simulink model "DiagCCaller_TestHarness"  (R2019a)
settings: Solver=FixedStepDiscrete  StartTime=0.0  StopTime=10.0  FixedStep=0.1  RelTol=1e-3  EnableMultiTasking=on
undefined symbols (not defined in the file): Dem_EventStatusType, sigbuilder_block
(part 2 of 4)

== system DiagCCaller_TestHarness/Debounce Enabled - RESET by Disable\Enable subsystem,Fault Active, FaultCnt = 10, PassCnt = -5, Heal 1  ==
  Bus Creator : BusCreator  Inputs=15
  Data Type Conversion{,1..2,9..14} (9 alike) : DataTypeConversion  OutDataTypeStr=boolean
  Data Type Conversion3 : DataTypeConversion  OutDataTypeStr=single
  Data Type Conversion4 : DataTypeConversion  OutDataTypeStr=single
  Data Type Conversion{5..8} (4 alike) : DataTypeConversion  OutDataTypeStr=int16
  Signal Builder : Subsystem  Tag=STV Subsys  LoadFcn=sigbuilder_block('load');  StartFcn=sigbuilder_block('start');  StopFcn=sigbuilder_block('stop');  ClipboardFcn=sigbuilder_block('clipboard');  TreatAsAtomicUnit=on  mask(Sigbuilder block){tuvar=[0:10]}
      mask help: Simulink:masks:SigbuilderBlock_MD
      mask init:
      | if ~strcmp(get_param(bdroot(gcbh),'SimulationStatus'),'stopped') tuvar = sigbuilder_block('maskInit'); end
      settings: CopyFcn=sigbuilder_block('copy');  DeleteFcn=sigbuilder_block('delete');  ModelCloseFcn=sigbuilder_block('modelClose');  PreSaveFcn=sigbuilder_block('preSave');  PauseFcn=sigbuilder_block('pause');  ContinueFcn=sigbuilder_block('continue');  NameChangeFcn=sigbuilder_block('namechange');  OpenFcn=sigbuilder_block('open',[5.4 30 1141.2 522.6 ]);  CloseFcn=sigbuilder_block('close');
      mask Display: plot(0, 0, 100, 100,[2, 2, 32, 32, 2], [68, 8, 8, 68, 68],[32, 2], [38, 38], [32, 19, 2],[53, 60, 44], [32, 17, 17, 2],[16, 16, 31, 31]);txt = getActiveGroup(gcbh);text(2, 100, txt,'verticalAlignment', 'top');
  Out1 : Outport
  wires:
  Bus Creator/1 -> Out1/1
  Signal Builder/2(DiagInput) -> Data Type Conversion1/1
  Signal Builder/3(StartupComp) -> Data Type Conversion2/1
  Signal Builder/4(MaxValue) -> Data Type Conversion4/1
  Signal Builder/5(MinValue) -> Data Type Conversion3/1
  Signal Builder/6(UpCount) -> Data Type Conversion5/1
  Signal Builder/7(DownCount) -> Data Type Conversion6/1
  Signal Builder/8(FaultCountThd) -> Data Type Conversion7/1
  Signal Builder/9(PassCountThd) -> Data Type Conversion8/1
  Signal Builder/10(DebounceEn) -> Data Type Conversion9/1
  Signal Builder/11(DiagReset) -> Data Type Conversion10/1
  Signal Builder/12(DiagEnable) -> Data Type Conversion11/1
  Signal Builder/13(HealEnable) -> Data Type Conversion12/1
  Signal Builder/14(PreestorageFreezeTrigger) -> Data Type Conversion13/1
  Signal Builder/15(JumpDownEn) -> Data Type Conversion14/1
  Signal Builder/1(EnableSubsystem) -> Data Type Conversion/1
  Data Type Conversion/1 -> Bus Creator/1  "EnableSubsystem"
  Data Type Conversion1/1 -> Bus Creator/2  "DiagInput"
  Data Type Conversion2/1 -> Bus Creator/3  "StartupComp"
  Data Type Conversion4/1 -> Bus Creator/4  "MaxValue"
  Data Type Conversion3/1 -> Bus Creator/5  "MinValue"
  Data Type Conversion5/1 -> Bus Creator/6  "UpCount"
  Data Type Conversion6/1 -> Bus Creator/7  "DownCount"
  Data Type Conversion7/1 -> Bus Creator/8  "FaultCountThd"
  Data Type Conversion8/1 -> Bus Creator/9  "PassCountThd"
  Data Type Conversion9/1 -> Bus Creator/10  "DebounceEn"
  Data Type Conversion10/1 -> Bus Creator/11  "DiagReset"
  Data Type Conversion11/1 -> Bus Creator/12  "DiagEnable"
  Data Type Conversion12/1 -> Bus Creator/13  "HealEnable"
  Data Type Conversion13/1 -> Bus Creator/14  "PreestorageFreezeTrigger"
  Data Type Conversion14/1 -> Bus Creator/15  "JumpDownEn"

== system DiagCCaller_TestHarness/Debounce Enabled - RESET by Disable\Enable subsystem,Fault Active, FaultCnt = 10, PassCnt = 0 , Heal 0  ==
  Bus Creator : BusCreator  Inputs=15
  Data Type Conversion{,1..2,9..14} (9 alike) : DataTypeConversion  OutDataTypeStr=boolean
  Data Type Conversion3 : DataTypeConversion  OutDataTypeStr=single
  Data Type Conversion4 : DataTypeConversion  OutDataTypeStr=single
  Data Type Conversion{5..8} (4 alike) : DataTypeConversion  OutDataTypeStr=int16
  Signal Builder : Subsystem  Tag=STV Subsys  LoadFcn=sigbuilder_block('load');  StartFcn=sigbuilder_block('start');  StopFcn=sigbuilder_block('stop');  ClipboardFcn=sigbuilder_block('clipboard');  TreatAsAtomicUnit=on  mask(Sigbuilder block){tuvar=[0:10]}
      mask help: Simulink:masks:SigbuilderBlock_MD
      mask init:
      | if ~strcmp(get_param(bdroot(gcbh),'SimulationStatus'),'stopped') tuvar = sigbuilder_block('maskInit'); end
      settings: CopyFcn=sigbuilder_block('copy');  DeleteFcn=sigbuilder_block('delete');  ModelCloseFcn=sigbuilder_block('modelClose');  PreSaveFcn=sigbuilder_block('preSave');  PauseFcn=sigbuilder_block('pause');  ContinueFcn=sigbuilder_block('continue');  NameChangeFcn=sigbuilder_block('namechange');  OpenFcn=sigbuilder_block('open',[5.4 5.4 1141.2 580.8 ]);  CloseFcn=sigbuilder_block('close');
      mask Display: plot(0, 0, 100, 100,[2, 2, 32, 32, 2], [68, 8, 8, 68, 68],[32, 2], [38, 38], [32, 19, 2],[53, 60, 44], [32, 17, 17, 2],[16, 16, 31, 31]);txt = getActiveGroup(gcbh);text(2, 100, txt,'verticalAlignment', 'top');
  Out1 : Outport
  wires:
  Data Type Conversion14/1 -> Bus Creator/15  "JumpDownEn"
  Data Type Conversion13/1 -> Bus Creator/14  "PreestorageFreezeTrigger"
  Data Type Conversion12/1 -> Bus Creator/13  "HealEnable"
  Data Type Conversion11/1 -> Bus Creator/12  "DiagEnable"
  Data Type Conversion10/1 -> Bus Creator/11  "DiagReset"
  Data Type Conversion9/1 -> Bus Creator/10  "DebounceEn"
  Data Type Conversion8/1 -> Bus Creator/9  "PassCountThd"
  Data Type Conversion7/1 -> Bus Creator/8  "FaultCountThd"
  Data Type Conversion6/1 -> Bus Creator/7  "DownCount"
  Data Type Conversion5/1 -> Bus Creator/6  "UpCount"
  Data Type Conversion3/1 -> Bus Creator/5  "MinValue"
  Data Type Conversion4/1 -> Bus Creator/4  "MaxValue"
  Data Type Conversion2/1 -> Bus Creator/3  "StartupComp"
  Data Type Conversion1/1 -> Bus Creator/2  "DiagInput"
  Data Type Conversion/1 -> Bus Creator/1  "EnableSubsystem"
  Signal Builder/1(EnableSubsystem) -> Data Type Conversion/1
  Signal Builder/15(JumpDownEn) -> Data Type Conversion14/1
  Signal Builder/14(PreestorageFreezeTrigger) -> Data Type Conversion13/1
  Signal Builder/13(HealEnable) -> Data Type Conversion12/1
  Signal Builder/12(DiagEnable) -> Data Type Conversion11/1
  Signal Builder/11(DiagReset) -> Data Type Conversion10/1
  Signal Builder/10(DebounceEn) -> Data Type Conversion9/1
  Signal Builder/9(PassCountThd) -> Data Type Conversion8/1
  Signal Builder/8(FaultCountThd) -> Data Type Conversion7/1
  Signal Builder/7(DownCount) -> Data Type Conversion6/1
  Signal Builder/6(UpCount) -> Data Type Conversion5/1
  Signal Builder/5(MinValue) -> Data Type Conversion3/1
  Signal Builder/4(MaxValue) -> Data Type Conversion4/1
  Signal Builder/3(StartupComp) -> Data Type Conversion2/1
  Signal Builder/2(DiagInput) -> Data Type Conversion1/1
  Bus Creator/1 -> Out1/1

== system DiagCCaller_TestHarness/Debounce Enabled - RESET by Disable\Enable subsystem,Fault Inactive,  FaultCnt = 10, PassCnt = -5 , Heal 1  ==
  Bus Creator : BusCreator  Inputs=15
  Data Type Conversion{,1..2,9..14} (9 alike) : DataTypeConversion  OutDataTypeStr=boolean
  Data Type Conversion3 : DataTypeConversion  OutDataTypeStr=single
  Data Type Conversion4 : DataTypeConversion  OutDataTypeStr=single
  Data Type Conversion{5..8} (4 alike) : DataTypeConversion  OutDataTypeStr=int16
  Signal Builder : Subsystem  Tag=STV Subsys  LoadFcn=sigbuilder_block('load');  StartFcn=sigbuilder_block('start');  StopFcn=sigbuilder_block('stop');  ClipboardFcn=sigbuilder_block('clipboard');  TreatAsAtomicUnit=on  mask(Sigbuilder block){tuvar=[0:10]}
      mask help: Simulink:masks:SigbuilderBlock_MD
      mask init:
      | if ~strcmp(get_param(bdroot(gcbh),'SimulationStatus'),'stopped') tuvar = sigbuilder_block('maskInit'); end
      settings: CopyFcn=sigbuilder_block('copy');  DeleteFcn=sigbuilder_block('delete');  ModelCloseFcn=sigbuilder_block('modelClose');  PreSaveFcn=sigbuilder_block('preSave');  PauseFcn=sigbuilder_block('pause');  ContinueFcn=sigbuilder_block('continue');  NameChangeFcn=sigbuilder_block('namechange');  OpenFcn=sigbuilder_block('open',[1440 -222 1440 813.6 ]);  CloseFcn=sigbuilder_block('close');
      mask Display: plot(0, 0, 100, 100,[2, 2, 32, 32, 2], [68, 8, 8, 68, 68],[32, 2], [38, 38], [32, 19, 2],[53, 60, 44], [32, 17, 17, 2],[16, 16, 31, 31]);txt = getActiveGroup(gcbh);text(2, 100, txt,'verticalAlignment', 'top');
  Out1 : Outport
  wires:
  Data Type Conversion14/1 -> Bus Creator/15  "JumpDownEn"
  Data Type Conversion13/1 -> Bus Creator/14  "PreestorageFreezeTrigger"
  Data Type Conversion12/1 -> Bus Creator/13  "HealEnable"
  Data Type Conversion11/1 -> Bus Creator/12  "DiagEnable"
  Data Type Conversion10/1 -> Bus Creator/11  "DiagReset"
  Data Type Conversion9/1 -> Bus Creator/10  "DebounceEn"
  Data Type Conversion8/1 -> Bus Creator/9  "PassCountThd"
  Data Type Conversion7/1 -> Bus Creator/8  "FaultCountThd"
  Data Type Conversion6/1 -> Bus Creator/7  "DownCount"
  Data Type Conversion5/1 -> Bus Creator/6  "UpCount"
  Data Type Conversion3/1 -> Bus Creator/5  "MinValue"
  Data Type Conversion4/1 -> Bus Creator/4  "MaxValue"
  Data Type Conversion2/1 -> Bus Creator/3  "StartupComp"
  Data Type Conversion1/1 -> Bus Creator/2  "DiagInput"
  Data Type Conversion/1 -> Bus Creator/1  "EnableSubsystem"
  Signal Builder/1(EnableSubsystem) -> Data Type Conversion/1
  Signal Builder/15(JumpDownEn) -> Data Type Conversion14/1
  Signal Builder/14(PreestorageFreezeTrigger) -> Data Type Conversion13/1
  Signal Builder/13(HealEnable) -> Data Type Conversion12/1
  Signal Builder/12(DiagEnable) -> Data Type Conversion11/1
  Signal Builder/11(DiagReset) -> Data Type Conversion10/1
  Signal Builder/10(DebounceEn) -> Data Type Conversion9/1
  Signal Builder/9(PassCountThd) -> Data Type Conversion8/1
  Signal Builder/8(FaultCountThd) -> Data Type Conversion7/1
  Signal Builder/7(DownCount) -> Data Type Conversion6/1
  Signal Builder/6(UpCount) -> Data Type Conversion5/1
  Signal Builder/5(MinValue) -> Data Type Conversion3/1
  Signal Builder/4(MaxValue) -> Data Type Conversion4/1
  Signal Builder/3(StartupComp) -> Data Type Conversion2/1
  Signal Builder/2(DiagInput) -> Data Type Conversion1/1
  Bus Creator/1 -> Out1/1

== system DiagCCaller_TestHarness/Debounce Enabled - RESET by Disable\Enable subsystem,Fault Inactive, , FaultCnt = 10, PassCnt = 0 , Heal 0  ==
  Bus Creator : BusCreator  Inputs=15
  Data Type Conversion{,1..2,9..14} (9 alike) : DataTypeConversion  OutDataTypeStr=boolean
  Data Type Conversion3 : DataTypeConversion  OutDataTypeStr=single
  Data Type Conversion4 : DataTypeConversion  OutDataTypeStr=single
  Data Type Conversion{5..8} (4 alike) : DataTypeConversion  OutDataTypeStr=int16
  Signal Builder : Subsystem  Tag=STV Subsys  LoadFcn=sigbuilder_block('load');  StartFcn=sigbuilder_block('start');  StopFcn=sigbuilder_block('stop');  ClipboardFcn=sigbuilder_block('clipboard');  TreatAsAtomicUnit=on  mask(Sigbuilder block){tuvar=[0:10]}
      mask help: Simulink:masks:SigbuilderBlock_MD
      mask init:
      | if ~strcmp(get_param(bdroot(gcbh),'SimulationStatus'),'stopped') tuvar = sigbuilder_block('maskInit'); end
      settings: CopyFcn=sigbuilder_block('copy');  DeleteFcn=sigbuilder_block('delete');  ModelCloseFcn=sigbuilder_block('modelClose');  PreSaveFcn=sigbuilder_block('preSave');  PauseFcn=sigbuilder_block('pause');  ContinueFcn=sigbuilder_block('continue');  NameChangeFcn=sigbuilder_block('namechange');  OpenFcn=sigbuilder_block('open',[5.4 30 1141.2 522.6 ]);  CloseFcn=sigbuilder_block('close');
      mask Display: plot(0, 0, 100, 100,[2, 2, 32, 32, 2], [68, 8, 8, 68, 68],[32, 2], [38, 38], [32, 19, 2],[53, 60, 44], [32, 17, 17, 2],[16, 16, 31, 31]);txt = getActiveGroup(gcbh);text(2, 100, txt,'verticalAlignment', 'top');
  Out1 : Outport
  wires:
  Data Type Conversion14/1 -> Bus Creator/15  "JumpDownEn"
  Data Type Conversion13/1 -> Bus Creator/14  "PreestorageFreezeTrigger"
  Data Type Conversion12/1 -> Bus Creator/13  "HealEnable"
  Data Type Conversion11/1 -> Bus Creator/12  "DiagEnable"
  Data Type Conversion10/1 -> Bus Creator/11  "DiagReset"
  Data Type Conversion9/1 -> Bus Creator/10  "DebounceEn"
  Data Type Conversion8/1 -> Bus Creator/9  "PassCountThd"
  Data Type Conversion7/1 -> Bus Creator/8  "FaultCountThd"
  Data Type Conversion6/1 -> Bus Creator/7  "DownCount"
  Data Type Conversion5/1 -> Bus Creator/6  "UpCount"
  Data Type Conversion3/1 -> Bus Creator/5  "MinValue"
  Data Type Conversion4/1 -> Bus Creator/4  "MaxValue"
  Data Type Conversion2/1 -> Bus Creator/3  "StartupComp"
  Data Type Conversion1/1 -> Bus Creator/2  "DiagInput"
  Data Type Conversion/1 -> Bus Creator/1  "EnableSubsystem"
  Signal Builder/1(EnableSubsystem) -> Data Type Conversion/1
  Signal Builder/15(JumpDownEn) -> Data Type Conversion14/1
  Signal Builder/14(PreestorageFreezeTrigger) -> Data Type Conversion13/1
  Signal Builder/13(HealEnable) -> Data Type Conversion12/1
  Signal Builder/12(DiagEnable) -> Data Type Conversion11/1
  Signal Builder/11(DiagReset) -> Data Type Conversion10/1
  Signal Builder/10(DebounceEn) -> Data Type Conversion9/1
  Signal Builder/9(PassCountThd) -> Data Type Conversion8/1
  Signal Builder/8(FaultCountThd) -> Data Type Conversion7/1
  Signal Builder/7(DownCount) -> Data Type Conversion6/1
  Signal Builder/6(UpCount) -> Data Type Conversion5/1
  Signal Builder/5(MinValue) -> Data Type Conversion3/1
  Signal Builder/4(MaxValue) -> Data Type Conversion4/1
  Signal Builder/3(StartupComp) -> Data Type Conversion2/1
  Signal Builder/2(DiagInput) -> Data Type Conversion1/1
  Bus Creator/1 -> Out1/1

== system DiagCCaller_TestHarness/Debounce Enabled - RESET by Disable\Enable subsystem,Fault Inactive, , FaultCnt = 10, PassCnt = 0 , Heal 0 1 ==
  Bus Creator : BusCreator  Inputs=15
  Data Type Conversion{,1..2,9..14} (9 alike) : DataTypeConversion  OutDataTypeStr=boolean
  Data Type Conversion3 : DataTypeConversion  OutDataTypeStr=single
  Data Type Conversion4 : DataTypeConversion  OutDataTypeStr=single
  Data Type Conversion{5..8} (4 alike) : DataTypeConversion  OutDataTypeStr=int16
  Signal Builder : Subsystem  Tag=STV Subsys  LoadFcn=sigbuilder_block('load');  StartFcn=sigbuilder_block('start');  StopFcn=sigbuilder_block('stop');  ClipboardFcn=sigbuilder_block('clipboard');  TreatAsAtomicUnit=on  mask(Sigbuilder block){tuvar=[0:10]}
      mask help: Simulink:masks:SigbuilderBlock_MD
      mask init:
      | if ~strcmp(get_param(bdroot(gcbh),'SimulationStatus'),'stopped') tuvar = sigbuilder_block('maskInit'); end
      settings: CopyFcn=sigbuilder_block('copy');  DeleteFcn=sigbuilder_block('delete');  ModelCloseFcn=sigbuilder_block('modelClose');  PreSaveFcn=sigbuilder_block('preSave');  PauseFcn=sigbuilder_block('pause');  ContinueFcn=sigbuilder_block('continue');  NameChangeFcn=sigbuilder_block('namechange');  OpenFcn=sigbuilder_block('open',[5.4 30 1141.2 522.6 ]);  CloseFcn=sigbuilder_block('close');
      mask Display: plot(0, 0, 100, 100,[2, 2, 32, 32, 2], [68, 8, 8, 68, 68],[32, 2], [38, 38], [32, 19, 2],[53, 60, 44], [32, 17, 17, 2],[16, 16, 31, 31]);txt = getActiveGroup(gcbh);text(2, 100, txt,'verticalAlignment', 'top');
  Out1 : Outport
  wires:
  Bus Creator/1 -> Out1/1
  Signal Builder/2(DiagInput) -> Data Type Conversion1/1
  Signal Builder/3(StartupComp) -> Data Type Conversion2/1
  Signal Builder/4(MaxValue) -> Data Type Conversion4/1
  Signal Builder/5(MinValue) -> Data Type Conversion3/1
  Signal Builder/6(UpCount) -> Data Type Conversion5/1
  Signal Builder/7(DownCount) -> Data Type Conversion6/1
  Signal Builder/8(FaultCountThd) -> Data Type Conversion7/1
  Signal Builder/9(PassCountThd) -> Data Type Conversion8/1
  Signal Builder/10(DebounceEn) -> Data Type Conversion9/1
  Signal Builder/11(DiagReset) -> Data Type Conversion10/1
  Signal Builder/12(DiagEnable) -> Data Type Conversion11/1
  Signal Builder/13(HealEnable) -> Data Type Conversion12/1
  Signal Builder/14(PreestorageFreezeTrigger) -> Data Type Conversion13/1
  Signal Builder/15(JumpDownEn) -> Data Type Conversion14/1
  Signal Builder/1(EnableSubsystem) -> Data Type Conversion/1
  Data Type Conversion/1 -> Bus Creator/1  "EnableSubsystem"
  Data Type Conversion1/1 -> Bus Creator/2  "DiagInput"
  Data Type Conversion2/1 -> Bus Creator/3  "StartupComp"
  Data Type Conversion4/1 -> Bus Creator/4  "MaxValue"
  Data Type Conversion3/1 -> Bus Creator/5  "MinValue"
  Data Type Conversion5/1 -> Bus Creator/6  "UpCount"
  Data Type Conversion6/1 -> Bus Creator/7  "DownCount"
  Data Type Conversion7/1 -> Bus Creator/8  "FaultCountThd"
  Data Type Conversion8/1 -> Bus Creator/9  "PassCountThd"
  Data Type Conversion9/1 -> Bus Creator/10  "DebounceEn"
  Data Type Conversion10/1 -> Bus Creator/11  "DiagReset"
  Data Type Conversion11/1 -> Bus Creator/12  "DiagEnable"
  Data Type Conversion12/1 -> Bus Creator/13  "HealEnable"
  Data Type Conversion13/1 -> Bus Creator/14  "PreestorageFreezeTrigger"
  Data Type Conversion14/1 -> Bus Creator/15  "JumpDownEn"

== system DiagCCaller_TestHarness/Debounce Enabled - StartUpComp delay = 1s, Fault Active , FaultCnt = 10, PassCnt = -5 , Heal 1  ==
  Bus Creator : BusCreator  Inputs=15
  Data Type Conversion{,1..2,9..14} (9 alike) : DataTypeConversion  OutDataTypeStr=boolean
  Data Type Conversion3 : DataTypeConversion  OutDataTypeStr=single
  Data Type Conversion4 : DataTypeConversion  OutDataTypeStr=single
  Data Type Conversion{5..8} (4 alike) : DataTypeConversion  OutDataTypeStr=int16
  Signal Builder : Subsystem  Tag=STV Subsys  LoadFcn=sigbuilder_block('load');  StartFcn=sigbuilder_block('start');  StopFcn=sigbuilder_block('stop');  ClipboardFcn=sigbuilder_block('clipboard');  TreatAsAtomicUnit=on  mask(Sigbuilder block){tuvar=[0:10]}
      mask help: Simulink:masks:SigbuilderBlock_MD
      mask init:
      | if ~strcmp(get_param(bdroot(gcbh),'SimulationStatus'),'stopped') tuvar = sigbuilder_block('maskInit'); end
      settings: CopyFcn=sigbuilder_block('copy');  DeleteFcn=sigbuilder_block('delete');  ModelCloseFcn=sigbuilder_block('modelClose');  PreSaveFcn=sigbuilder_block('preSave');  PauseFcn=sigbuilder_block('pause');  ContinueFcn=sigbuilder_block('continue');  NameChangeFcn=sigbuilder_block('namechange');  OpenFcn=sigbuilder_block('open',[5.4 30 1141.2 522.6 ]);  CloseFcn=sigbuilder_block('close');
      mask Display: plot(0, 0, 100, 100,[2, 2, 32, 32, 2], [68, 8, 8, 68, 68],[32, 2], [38, 38], [32, 19, 2],[53, 60, 44], [32, 17, 17, 2],[16, 16, 31, 31]);txt = getActiveGroup(gcbh);text(2, 100, txt,'verticalAlignment', 'top');
  Out1 : Outport
  wires:
  Bus Creator/1 -> Out1/1
  Signal Builder/2(DiagInput) -> Data Type Conversion1/1
  Signal Builder/3(StartupComp) -> Data Type Conversion2/1
  Signal Builder/4(MaxValue) -> Data Type Conversion4/1
  Signal Builder/5(MinValue) -> Data Type Conversion3/1
  Signal Builder/6(UpCount) -> Data Type Conversion5/1
  Signal Builder/7(DownCount) -> Data Type Conversion6/1
  Signal Builder/8(FaultCountThd) -> Data Type Conversion7/1
  Signal Builder/9(PassCountThd) -> Data Type Conversion8/1
  Signal Builder/10(DebounceEn) -> Data Type Conversion9/1
  Signal Builder/11(DiagReset) -> Data Type Conversion10/1
  Signal Builder/12(DiagEnable) -> Data Type Conversion11/1
  Signal Builder/13(HealEnable) -> Data Type Conversion12/1
  Signal Builder/14(PreestorageFreezeTrigger) -> Data Type Conversion13/1
  Signal Builder/15(JumpDownEn) -> Data Type Conversion14/1
  Signal Builder/1(EnableSubsystem) -> Data Type Conversion/1
  Data Type Conversion/1 -> Bus Creator/1  "EnableSubsystem"
  Data Type Conversion1/1 -> Bus Creator/2  "DiagInput"
  Data Type Conversion2/1 -> Bus Creator/3  "StartupComp"
  Data Type Conversion4/1 -> Bus Creator/4  "MaxValue"
  Data Type Conversion3/1 -> Bus Creator/5  "MinValue"
  Data Type Conversion5/1 -> Bus Creator/6  "UpCount"
  Data Type Conversion6/1 -> Bus Creator/7  "DownCount"
  Data Type Conversion7/1 -> Bus Creator/8  "FaultCountThd"
  Data Type Conversion8/1 -> Bus Creator/9  "PassCountThd"
  Data Type Conversion9/1 -> Bus Creator/10  "DebounceEn"
  Data Type Conversion10/1 -> Bus Creator/11  "DiagReset"
  Data Type Conversion11/1 -> Bus Creator/12  "DiagEnable"
  Data Type Conversion12/1 -> Bus Creator/13  "HealEnable"
  Data Type Conversion13/1 -> Bus Creator/14  "PreestorageFreezeTrigger"
  Data Type Conversion14/1 -> Bus Creator/15  "JumpDownEn"

== system DiagCCaller_TestHarness/Debounce Enabled - StartUpComp delay = 1s, Fault Active , FaultCnt = 10, PassCnt = 0 , Heal 0  ==
  Bus Creator : BusCreator  Inputs=15
  Data Type Conversion{,1..2,9..14} (9 alike) : DataTypeConversion  OutDataTypeStr=boolean
  Data Type Conversion3 : DataTypeConversion  OutDataTypeStr=single
  Data Type Conversion4 : DataTypeConversion  OutDataTypeStr=single
  Data Type Conversion{5..8} (4 alike) : DataTypeConversion  OutDataTypeStr=int16
  Signal Builder : Subsystem  Tag=STV Subsys  LoadFcn=sigbuilder_block('load');  StartFcn=sigbuilder_block('start');  StopFcn=sigbuilder_block('stop');  ClipboardFcn=sigbuilder_block('clipboard');  TreatAsAtomicUnit=on  mask(Sigbuilder block){tuvar=[0:10]}
      mask help: Simulink:masks:SigbuilderBlock_MD
      mask init:
      | if ~strcmp(get_param(bdroot(gcbh),'SimulationStatus'),'stopped') tuvar = sigbuilder_block('maskInit'); end
      settings: CopyFcn=sigbuilder_block('copy');  DeleteFcn=sigbuilder_block('delete');  ModelCloseFcn=sigbuilder_block('modelClose');  PreSaveFcn=sigbuilder_block('preSave');  PauseFcn=sigbuilder_block('pause');  ContinueFcn=sigbuilder_block('continue');  NameChangeFcn=sigbuilder_block('namechange');  OpenFcn=sigbuilder_block('open',[5.4 30 1141.2 522.6 ]);  CloseFcn=sigbuilder_block('close');
      mask Display: plot(0, 0, 100, 100,[2, 2, 32, 32, 2], [68, 8, 8, 68, 68],[32, 2], [38, 38], [32, 19, 2],[53, 60, 44], [32, 17, 17, 2],[16, 16, 31, 31]);txt = getActiveGroup(gcbh);text(2, 100, txt,'verticalAlignment', 'top');
  Out1 : Outport
  wires:
  Data Type Conversion14/1 -> Bus Creator/15  "JumpDownEn"
  Data Type Conversion13/1 -> Bus Creator/14  "PreestorageFreezeTrigger"
  Data Type Conversion12/1 -> Bus Creator/13  "HealEnable"
  Data Type Conversion11/1 -> Bus Creator/12  "DiagEnable"
  Data Type Conversion10/1 -> Bus Creator/11  "DiagReset"
  Data Type Conversion9/1 -> Bus Creator/10  "DebounceEn"
  Data Type Conversion8/1 -> Bus Creator/9  "PassCountThd"
  Data Type Conversion7/1 -> Bus Creator/8  "FaultCountThd"
  Data Type Conversion6/1 -> Bus Creator/7  "DownCount"
  Data Type Conversion5/1 -> Bus Creator/6  "UpCount"
  Data Type Conversion3/1 -> Bus Creator/5  "MinValue"
  Data Type Conversion4/1 -> Bus Creator/4  "MaxValue"
  Data Type Conversion2/1 -> Bus Creator/3  "StartupComp"
  Data Type Conversion1/1 -> Bus Creator/2  "DiagInput"
  Data Type Conversion/1 -> Bus Creator/1  "EnableSubsystem"
  Signal Builder/1(EnableSubsystem) -> Data Type Conversion/1
  Signal Builder/15(JumpDownEn) -> Data Type Conversion14/1
  Signal Builder/14(PreestorageFreezeTrigger) -> Data Type Conversion13/1
  Signal Builder/13(HealEnable) -> Data Type Conversion12/1
  Signal Builder/12(DiagEnable) -> Data Type Conversion11/1
  Signal Builder/11(DiagReset) -> Data Type Conversion10/1
  Signal Builder/10(DebounceEn) -> Data Type Conversion9/1
  Signal Builder/9(PassCountThd) -> Data Type Conversion8/1
  Signal Builder/8(FaultCountThd) -> Data Type Conversion7/1
  Signal Builder/7(DownCount) -> Data Type Conversion6/1
  Signal Builder/6(UpCount) -> Data Type Conversion5/1
  Signal Builder/5(MinValue) -> Data Type Conversion3/1
  Signal Builder/4(MaxValue) -> Data Type Conversion4/1
  Signal Builder/3(StartupComp) -> Data Type Conversion2/1
  Signal Builder/2(DiagInput) -> Data Type Conversion1/1
  Bus Creator/1 -> Out1/1

== system DiagCCaller_TestHarness/Debounce Enabled - StartUpComp delay = 1s, Fault Inactive , FaultCnt = 10, PassCnt = -5, Heal 1  ==
  Bus Creator : BusCreator  Inputs=15
  Data Type Conversion{,1..2,9..14} (9 alike) : DataTypeConversion  OutDataTypeStr=boolean
  Data Type Conversion3 : DataTypeConversion  OutDataTypeStr=single
  Data Type Conversion4 : DataTypeConversion  OutDataTypeStr=single
  Data Type Conversion{5..8} (4 alike) : DataTypeConversion  OutDataTypeStr=int16
  Signal Builder : Subsystem  Tag=STV Subsys  LoadFcn=sigbuilder_block('load');  StartFcn=sigbuilder_block('start');  StopFcn=sigbuilder_block('stop');  ClipboardFcn=sigbuilder_block('clipboard');  TreatAsAtomicUnit=on  mask(Sigbuilder block){tuvar=[0:10]}
      mask help: Simulink:masks:SigbuilderBlock_MD
      mask init:
      | if ~strcmp(get_param(bdroot(gcbh),'SimulationStatus'),'stopped') tuvar = sigbuilder_block('maskInit'); end
      settings: CopyFcn=sigbuilder_block('copy');  DeleteFcn=sigbuilder_block('delete');  ModelCloseFcn=sigbuilder_block('modelClose');  PreSaveFcn=sigbuilder_block('preSave');  PauseFcn=sigbuilder_block('pause');  ContinueFcn=sigbuilder_block('continue');  NameChangeFcn=sigbuilder_block('namechange');  OpenFcn=sigbuilder_block('open',[5.4 30 1141.2 522.6 ]);  CloseFcn=sigbuilder_block('close');
      mask Display: plot(0, 0, 100, 100,[2, 2, 32, 32, 2], [68, 8, 8, 68, 68],[32, 2], [38, 38], [32, 19, 2],[53, 60, 44], [32, 17, 17, 2],[16, 16, 31, 31]);txt = getActiveGroup(gcbh);text(2, 100, txt,'verticalAlignment', 'top');
  Out1 : Outport
  wires:
  Data Type Conversion14/1 -> Bus Creator/15  "JumpDownEn"
  Data Type Conversion13/1 -> Bus Creator/14  "PreestorageFreezeTrigger"
  Data Type Conversion12/1 -> Bus Creator/13  "HealEnable"
  Data Type Conversion11/1 -> Bus Creator/12  "DiagEnable"
  Data Type Conversion10/1 -> Bus Creator/11  "DiagReset"
  Data Type Conversion9/1 -> Bus Creator/10  "DebounceEn"
  Data Type Conversion8/1 -> Bus Creator/9  "PassCountThd"
  Data Type Conversion7/1 -> Bus Creator/8  "FaultCountThd"
  Data Type Conversion6/1 -> Bus Creator/7  "DownCount"
  Data Type Conversion5/1 -> Bus Creator/6  "UpCount"
  Data Type Conversion3/1 -> Bus Creator/5  "MinValue"
  Data Type Conversion4/1 -> Bus Creator/4  "MaxValue"
  Data Type Conversion2/1 -> Bus Creator/3  "StartupComp"
  Data Type Conversion1/1 -> Bus Creator/2  "DiagInput"
  Data Type Conversion/1 -> Bus Creator/1  "EnableSubsystem"
  Signal Builder/1(EnableSubsystem) -> Data Type Conversion/1
  Signal Builder/15(JumpDownEn) -> Data Type Conversion14/1
  Signal Builder/14(PreestorageFreezeTrigger) -> Data Type Conversion13/1
  Signal Builder/13(HealEnable) -> Data Type Conversion12/1
  Signal Builder/12(DiagEnable) -> Data Type Conversion11/1
  Signal Builder/11(DiagReset) -> Data Type Conversion10/1
  Signal Builder/10(DebounceEn) -> Data Type Conversion9/1
  Signal Builder/9(PassCountThd) -> Data Type Conversion8/1
  Signal Builder/8(FaultCountThd) -> Data Type Conversion7/1
  Signal Builder/7(DownCount) -> Data Type Conversion6/1
  Signal Builder/6(UpCount) -> Data Type Conversion5/1
  Signal Builder/5(MinValue) -> Data Type Conversion3/1
  Signal Builder/4(MaxValue) -> Data Type Conversion4/1
  Signal Builder/3(StartupComp) -> Data Type Conversion2/1
  Signal Builder/2(DiagInput) -> Data Type Conversion1/1
  Bus Creator/1 -> Out1/1

== system DiagCCaller_TestHarness/Debounce Enabled - StartUpComp delay = 1s, Fault Inactive , FaultCnt = 10, PassCnt = 0 , Heal 0  ==
  Bus Creator : BusCreator  Inputs=15
  Data Type Conversion{,1..2,9..14} (9 alike) : DataTypeConversion  OutDataTypeStr=boolean
  Data Type Conversion3 : DataTypeConversion  OutDataTypeStr=single
  Data Type Conversion4 : DataTypeConversion  OutDataTypeStr=single
  Data Type Conversion{5..8} (4 alike) : DataTypeConversion  OutDataTypeStr=int16
  Signal Builder : Subsystem  Tag=STV Subsys  LoadFcn=sigbuilder_block('load');  StartFcn=sigbuilder_block('start');  StopFcn=sigbuilder_block('stop');  ClipboardFcn=sigbuilder_block('clipboard');  TreatAsAtomicUnit=on  mask(Sigbuilder block){tuvar=[0:10]}
      mask help: Simulink:masks:SigbuilderBlock_MD
      mask init:
      | if ~strcmp(get_param(bdroot(gcbh),'SimulationStatus'),'stopped') tuvar = sigbuilder_block('maskInit'); end
      settings: CopyFcn=sigbuilder_block('copy');  DeleteFcn=sigbuilder_block('delete');  ModelCloseFcn=sigbuilder_block('modelClose');  PreSaveFcn=sigbuilder_block('preSave');  PauseFcn=sigbuilder_block('pause');  ContinueFcn=sigbuilder_block('continue');  NameChangeFcn=sigbuilder_block('namechange');  OpenFcn=sigbuilder_block('open',[5.4 30 1141.2 522.6 ]);  CloseFcn=sigbuilder_block('close');
      mask Display: plot(0, 0, 100, 100,[2, 2, 32, 32, 2], [68, 8, 8, 68, 68],[32, 2], [38, 38], [32, 19, 2],[53, 60, 44], [32, 17, 17, 2],[16, 16, 31, 31]);txt = getActiveGroup(gcbh);text(2, 100, txt,'verticalAlignment', 'top');
  Out1 : Outport
  wires:
  Bus Creator/1 -> Out1/1
  Signal Builder/2(DiagInput) -> Data Type Conversion1/1
  Signal Builder/3(StartupComp) -> Data Type Conversion2/1
  Signal Builder/4(MaxValue) -> Data Type Conversion4/1
  Signal Builder/5(MinValue) -> Data Type Conversion3/1
  Signal Builder/6(UpCount) -> Data Type Conversion5/1
  Signal Builder/7(DownCount) -> Data Type Conversion6/1
  Signal Builder/8(FaultCountThd) -> Data Type Conversion7/1
  Signal Builder/9(PassCountThd) -> Data Type Conversion8/1
  Signal Builder/10(DebounceEn) -> Data Type Conversion9/1
  Signal Builder/11(DiagReset) -> Data Type Conversion10/1
  Signal Builder/12(DiagEnable) -> Data Type Conversion11/1
  Signal Builder/13(HealEnable) -> Data Type Conversion12/1
  Signal Builder/14(PreestorageFreezeTrigger) -> Data Type Conversion13/1
  Signal Builder/15(JumpDownEn) -> Data Type Conversion14/1
  Signal Builder/1(EnableSubsystem) -> Data Type Conversion/1
  Data Type Conversion/1 -> Bus Creator/1  "EnableSubsystem"
  Data Type Conversion1/1 -> Bus Creator/2  "DiagInput"
  Data Type Conversion2/1 -> Bus Creator/3  "StartupComp"
  Data Type Conversion4/1 -> Bus Creator/4  "MaxValue"
  Data Type Conversion3/1 -> Bus Creator/5  "MinValue"
  Data Type Conversion5/1 -> Bus Creator/6  "UpCount"
  Data Type Conversion6/1 -> Bus Creator/7  "DownCount"
  Data Type Conversion7/1 -> Bus Creator/8  "FaultCountThd"
  Data Type Conversion8/1 -> Bus Creator/9  "PassCountThd"
  Data Type Conversion9/1 -> Bus Creator/10  "DebounceEn"
  Data Type Conversion10/1 -> Bus Creator/11  "DiagReset"
  Data Type Conversion11/1 -> Bus Creator/12  "DiagEnable"
  Data Type Conversion12/1 -> Bus Creator/13  "HealEnable"
  Data Type Conversion13/1 -> Bus Creator/14  "PreestorageFreezeTrigger"
  Data Type Conversion14/1 -> Bus Creator/15  "JumpDownEn"

== system DiagCCaller_TestHarness/DebounceDisabled - RESET by Calibration DiagReset  ==
  Bus Creator : BusCreator  Inputs=15
  Data Type Conversion{,1..2,9..14} (9 alike) : DataTypeConversion  OutDataTypeStr=boolean
  Data Type Conversion3 : DataTypeConversion  OutDataTypeStr=single
  Data Type Conversion4 : DataTypeConversion  OutDataTypeStr=single
  Data Type Conversion{5..8} (4 alike) : DataTypeConversion  OutDataTypeStr=int16
  Signal Builder : Subsystem  Tag=STV Subsys  LoadFcn=sigbuilder_block('load');  StartFcn=sigbuilder_block('start');  StopFcn=sigbuilder_block('stop');  ClipboardFcn=sigbuilder_block('clipboard');  TreatAsAtomicUnit=on  mask(Sigbuilder block){tuvar=[0:10]}
      mask help: Simulink:masks:SigbuilderBlock_MD
      mask init:
      | if ~strcmp(get_param(bdroot(gcbh),'SimulationStatus'),'stopped') tuvar = sigbuilder_block('maskInit'); end
      settings: CopyFcn=sigbuilder_block('copy');  DeleteFcn=sigbuilder_block('delete');  ModelCloseFcn=sigbuilder_block('modelClose');  PreSaveFcn=sigbuilder_block('preSave');  PauseFcn=sigbuilder_block('pause');  ContinueFcn=sigbuilder_block('continue');  NameChangeFcn=sigbuilder_block('namechange');  OpenFcn=sigbuilder_block('open',[5.4 30 1141.2 522.6 ]);  CloseFcn=sigbuilder_block('close');
      mask Display: plot(0, 0, 100, 100,[2, 2, 32, 32, 2], [68, 8, 8, 68, 68],[32, 2], [38, 38], [32, 19, 2],[53, 60, 44], [32, 17, 17, 2],[16, 16, 31, 31]);txt = getActiveGroup(gcbh);text(2, 100, txt,'verticalAlignment', 'top');
  Out1 : Outport
  wires:
  Data Type Conversion14/1 -> Bus Creator/15  "JumpDownEn"
  Data Type Conversion13/1 -> Bus Creator/14  "PreestorageFreezeTrigger"
  Data Type Conversion12/1 -> Bus Creator/13  "HealEnable"
  Data Type Conversion11/1 -> Bus Creator/12  "DiagEnable"
  Data Type Conversion10/1 -> Bus Creator/11  "DiagReset"
  Data Type Conversion9/1 -> Bus Creator/10  "DebounceEn"
  Data Type Conversion8/1 -> Bus Creator/9  "PassCountThd"
  Data Type Conversion7/1 -> Bus Creator/8  "FaultCountThd"
  Data Type Conversion6/1 -> Bus Creator/7  "DownCount"
  Data Type Conversion5/1 -> Bus Creator/6  "UpCount"
  Data Type Conversion3/1 -> Bus Creator/5  "MinValue"
  Data Type Conversion4/1 -> Bus Creator/4  "MaxValue"
  Data Type Conversion2/1 -> Bus Creator/3  "StartupComp"
  Data Type Conversion1/1 -> Bus Creator/2  "DiagInput"
  Data Type Conversion/1 -> Bus Creator/1  "EnableSubsystem"
  Signal Builder/1(EnableSubsystem) -> Data Type Conversion/1
  Signal Builder/15(JumpDownEn) -> Data Type Conversion14/1
  Signal Builder/14(PreestorageFreezeTrigger) -> Data Type Conversion13/1
  Signal Builder/13(HealEnable) -> Data Type Conversion12/1
  Signal Builder/12(DiagEnable) -> Data Type Conversion11/1
  Signal Builder/11(DiagReset) -> Data Type Conversion10/1
  Signal Builder/10(DebounceEn) -> Data Type Conversion9/1
  Signal Builder/9(PassCountThd) -> Data Type Conversion8/1
  Signal Builder/8(FaultCountThd) -> Data Type Conversion7/1
  Signal Builder/7(DownCount) -> Data Type Conversion6/1
  Signal Builder/6(UpCount) -> Data Type Conversion5/1
  Signal Builder/5(MinValue) -> Data Type Conversion3/1
  Signal Builder/4(MaxValue) -> Data Type Conversion4/1
  Signal Builder/3(StartupComp) -> Data Type Conversion2/1
  Signal Builder/2(DiagInput) -> Data Type Conversion1/1
  Bus Creator/1 -> Out1/1

== system DiagCCaller_TestHarness/DebounceDisabled - RESET by Disable\Enable subsystem  ==
  Bus Creator : BusCreator  Inputs=15
  Data Type Conversion{,1..2,9..14} (9 alike) : DataTypeConversion  OutDataTypeStr=boolean
  Data Type Conversion3 : DataTypeConversion  OutDataTypeStr=single
  Data Type Conversion4 : DataTypeConversion  OutDataTypeStr=single
  Data Type Conversion{5..8} (4 alike) : DataTypeConversion  OutDataTypeStr=int16
  Signal Builder : Subsystem  Tag=STV Subsys  LoadFcn=sigbuilder_block('load');  StartFcn=sigbuilder_block('start');  StopFcn=sigbuilder_block('stop');  ClipboardFcn=sigbuilder_block('clipboard');  TreatAsAtomicUnit=on  mask(Sigbuilder block){tuvar=[0:10]}
      mask help: Simulink:masks:SigbuilderBlock_MD
      mask init:
      | if ~strcmp(get_param(bdroot(gcbh),'SimulationStatus'),'stopped') tuvar = sigbuilder_block('maskInit'); end
      settings: CopyFcn=sigbuilder_block('copy');  DeleteFcn=sigbuilder_block('delete');  ModelCloseFcn=sigbuilder_block('modelClose');  PreSaveFcn=sigbuilder_block('preSave');  PauseFcn=sigbuilder_block('pause');  ContinueFcn=sigbuilder_block('continue');  NameChangeFcn=sigbuilder_block('namechange');  OpenFcn=sigbuilder_block('open',[0 30 1152 561.6 ]);  CloseFcn=sigbuilder_block('close');
      mask Display: plot(0, 0, 100, 100,[2, 2, 32, 32, 2], [68, 8, 8, 68, 68],[32, 2], [38, 38], [32, 19, 2],[53, 60, 44], [32, 17, 17, 2],[16, 16, 31, 31]);txt = getActiveGroup(gcbh);text(2, 100, txt,'verticalAlignment', 'top');
  Out1 : Outport
  wires:
  Data Type Conversion14/1 -> Bus Creator/15  "JumpDownEn"
  Data Type Conversion13/1 -> Bus Creator/14  "PreestorageFreezeTrigger"
  Data Type Conversion12/1 -> Bus Creator/13  "HealEnable"
  Data Type Conversion11/1 -> Bus Creator/12  "DiagEnable"
  Data Type Conversion10/1 -> Bus Creator/11  "DiagReset"
  Data Type Conversion9/1 -> Bus Creator/10  "DebounceEn"
  Data Type Conversion8/1 -> Bus Creator/9  "PassCountThd"
  Data Type Conversion7/1 -> Bus Creator/8  "FaultCountThd"
  Data Type Conversion6/1 -> Bus Creator/7  "DownCount"
  Data Type Conversion5/1 -> Bus Creator/6  "UpCount"
  Data Type Conversion3/1 -> Bus Creator/5  "MinValue"
  Data Type Conversion4/1 -> Bus Creator/4  "MaxValue"
  Data Type Conversion2/1 -> Bus Creator/3  "StartupComp"
  Data Type Conversion1/1 -> Bus Creator/2  "DiagInput"
  Data Type Conversion/1 -> Bus Creator/1  "EnableSubsystem"
  Signal Builder/1(EnableSubsystem) -> Data Type Conversion/1
  Signal Builder/15(JumpDownEn) -> Data Type Conversion14/1
  Signal Builder/14(PreestorageFreezeTrigger) -> Data Type Conversion13/1
  Signal Builder/13(HealEnable) -> Data Type Conversion12/1
  Signal Builder/12(DiagEnable) -> Data Type Conversion11/1
  Signal Builder/11(DiagReset) -> Data Type Conversion10/1
  Signal Builder/10(DebounceEn) -> Data Type Conversion9/1
  Signal Builder/9(PassCountThd) -> Data Type Conversion8/1
  Signal Builder/8(FaultCountThd) -> Data Type Conversion7/1
  Signal Builder/7(DownCount) -> Data Type Conversion6/1
  Signal Builder/6(UpCount) -> Data Type Conversion5/1
  Signal Builder/5(MinValue) -> Data Type Conversion3/1
  Signal Builder/4(MaxValue) -> Data Type Conversion4/1
  Signal Builder/3(StartupComp) -> Data Type Conversion2/1
  Signal Builder/2(DiagInput) -> Data Type Conversion1/1
  Bus Creator/1 -> Out1/1

== system DiagCCaller_TestHarness/DebounceDisabled INIT Fault Active  ==
  Bus Creator : BusCreator  Inputs=15
  Data Type Conversion{,1..2,9..14} (9 alike) : DataTypeConversion  OutDataTypeStr=boolean
  Data Type Conversion3 : DataTypeConversion  OutDataTypeStr=single
  Data Type Conversion4 : DataTypeConversion  OutDataTypeStr=single
  Data Type Conversion{5..8} (4 alike) : DataTypeConversion  OutDataTypeStr=int16
  Signal Builder : Subsystem  Tag=STV Subsys  LoadFcn=sigbuilder_block('load');  StartFcn=sigbuilder_block('start');  StopFcn=sigbuilder_block('stop');  ClipboardFcn=sigbuilder_block('clipboard');  TreatAsAtomicUnit=on  mask(Sigbuilder block){tuvar=[0:10]}
      mask help: Simulink:masks:SigbuilderBlock_MD
      mask init:
      | if ~strcmp(get_param(bdroot(gcbh),'SimulationStatus'),'stopped') tuvar = sigbuilder_block('maskInit'); end
      settings: CopyFcn=sigbuilder_block('copy');  DeleteFcn=sigbuilder_block('delete');  ModelCloseFcn=sigbuilder_block('modelClose');  PreSaveFcn=sigbuilder_block('preSave');  PauseFcn=sigbuilder_block('pause');  ContinueFcn=sigbuilder_block('continue');  NameChangeFcn=sigbuilder_block('namechange');  OpenFcn=sigbuilder_block('open',[0 30 1152 561.6 ]);  CloseFcn=sigbuilder_block('close');
      mask Display: plot(0, 0, 100, 100,[2, 2, 32, 32, 2], [68, 8, 8, 68, 68],[32, 2], [38, 38], [32, 19, 2],[53, 60, 44], [32, 17, 17, 2],[16, 16, 31, 31]);txt = getActiveGroup(gcbh);text(2, 100, txt,'verticalAlignment', 'top');
  Out1 : Outport
  wires:
  Data Type Conversion14/1 -> Bus Creator/15  "JumpDownEn"
  Data Type Conversion13/1 -> Bus Creator/14  "PreestorageFreezeTrigger"
  Data Type Conversion12/1 -> Bus Creator/13  "HealEnable"
  Data Type Conversion11/1 -> Bus Creator/12  "DiagEnable"
  Data Type Conversion10/1 -> Bus Creator/11  "DiagReset"
  Data Type Conversion9/1 -> Bus Creator/10  "DebounceEn"
  Data Type Conversion8/1 -> Bus Creator/9  "PassCountThd"
  Data Type Conversion7/1 -> Bus Creator/8  "FaultCountThd"
  Data Type Conversion6/1 -> Bus Creator/7  "DownCount"
  Data Type Conversion5/1 -> Bus Creator/6  "UpCount"
  Data Type Conversion3/1 -> Bus Creator/5  "MinValue"
  Data Type Conversion4/1 -> Bus Creator/4  "MaxValue"
  Data Type Conversion2/1 -> Bus Creator/3  "StartupComp"
  Data Type Conversion1/1 -> Bus Creator/2  "DiagInput"
  Data Type Conversion/1 -> Bus Creator/1  "EnableSubsystem"
  Signal Builder/1(EnableSubsystem) -> Data Type Conversion/1
  Signal Builder/15(JumpDownEn) -> Data Type Conversion14/1
  Signal Builder/14(PreestorageFreezeTrigger) -> Data Type Conversion13/1
  Signal Builder/13(HealEnable) -> Data Type Conversion12/1
  Signal Builder/12(DiagEnable) -> Data Type Conversion11/1
  Signal Builder/11(DiagReset) -> Data Type Conversion10/1
  Signal Builder/10(DebounceEn) -> Data Type Conversion9/1
  Signal Builder/9(PassCountThd) -> Data Type Conversion8/1
  Signal Builder/8(FaultCountThd) -> Data Type Conversion7/1
  Signal Builder/7(DownCount) -> Data Type Conversion6/1
  Signal Builder/6(UpCount) -> Data Type Conversion5/1
  Signal Builder/5(MinValue) -> Data Type Conversion3/1
  Signal Builder/4(MaxValue) -> Data Type Conversion4/1
  Signal Builder/3(StartupComp) -> Data Type Conversion2/1
  Signal Builder/2(DiagInput) -> Data Type Conversion1/1
  Bus Creator/1 -> Out1/1

== system DiagCCaller_TestHarness/DebounceDisabled INIT Fault Inactive  ==
  Bus Creator : BusCreator  Inputs=15
  Data Type Conversion{,1..2,9..14} (9 alike) : DataTypeConversion  OutDataTypeStr=boolean
  Data Type Conversion3 : DataTypeConversion  OutDataTypeStr=single
  Data Type Conversion4 : DataTypeConversion  OutDataTypeStr=single
  Data Type Conversion{5..8} (4 alike) : DataTypeConversion  OutDataTypeStr=int16
  Signal Builder : Subsystem  Tag=STV Subsys  LoadFcn=sigbuilder_block('load');  StartFcn=sigbuilder_block('start');  StopFcn=sigbuilder_block('stop');  ClipboardFcn=sigbuilder_block('clipboard');  TreatAsAtomicUnit=on  mask(Sigbuilder block){tuvar=[0:10]}
      mask help: Simulink:masks:SigbuilderBlock_MD
      mask init:
      | if ~strcmp(get_param(bdroot(gcbh),'SimulationStatus'),'stopped') tuvar = sigbuilder_block('maskInit'); end
      settings: CopyFcn=sigbuilder_block('copy');  DeleteFcn=sigbuilder_block('delete');  ModelCloseFcn=sigbuilder_block('modelClose');  PreSaveFcn=sigbuilder_block('preSave');  PauseFcn=sigbuilder_block('pause');  ContinueFcn=sigbuilder_block('continue');  NameChangeFcn=sigbuilder_block('namechange');  OpenFcn=sigbuilder_block('open',[5.4 -26.4 1141.2 483.6 ]);  CloseFcn=sigbuilder_block('close');
      mask Display: plot(0, 0, 100, 100,[2, 2, 32, 32, 2], [68, 8, 8, 68, 68],[32, 2], [38, 38], [32, 19, 2],[53, 60, 44], [32, 17, 17, 2],[16, 16, 31, 31]);txt = getActiveGroup(gcbh);text(2, 100, txt,'verticalAlignment', 'top');
  Out1 : Outport
  wires:
  Bus Creator/1 -> Out1/1
  Signal Builder/2(DiagInput) -> Data Type Conversion1/1
  Signal Builder/3(StartupComp) -> Data Type Conversion2/1
  Signal Builder/4(MaxValue) -> Data Type Conversion4/1
  Signal Builder/5(MinValue) -> Data Type Conversion3/1
  Signal Builder/6(UpCount) -> Data Type Conversion5/1
  Signal Builder/7(DownCount) -> Data Type Conversion6/1
  Signal Builder/8(FaultCountThd) -> Data Type Conversion7/1
  Signal Builder/9(PassCountThd) -> Data Type Conversion8/1
  Signal Builder/10(DebounceEn) -> Data Type Conversion9/1
  Signal Builder/11(DiagReset) -> Data Type Conversion10/1
  Signal Builder/12(DiagEnable) -> Data Type Conversion11/1
  Signal Builder/13(HealEnable) -> Data Type Conversion12/1
  Signal Builder/14(PreestorageFreezeTrigger) -> Data Type Conversion13/1
  Signal Builder/15(JumpDownEn) -> Data Type Conversion14/1
  Signal Builder/1(EnableSubsystem) -> Data Type Conversion/1
  Data Type Conversion/1 -> Bus Creator/1  "EnableSubsystem"
  Data Type Conversion1/1 -> Bus Creator/2  "DiagInput"
  Data Type Conversion2/1 -> Bus Creator/3  "StartupComp"
  Data Type Conversion4/1 -> Bus Creator/4  "MaxValue"
  Data Type Conversion3/1 -> Bus Creator/5  "MinValue"
  Data Type Conversion5/1 -> Bus Creator/6  "UpCount"
  Data Type Conversion6/1 -> Bus Creator/7  "DownCount"
  Data Type Conversion7/1 -> Bus Creator/8  "FaultCountThd"
  Data Type Conversion8/1 -> Bus Creator/9  "PassCountThd"
  Data Type Conversion9/1 -> Bus Creator/10  "DebounceEn"
  Data Type Conversion10/1 -> Bus Creator/11  "DiagReset"
  Data Type Conversion11/1 -> Bus Creator/12  "DiagEnable"
  Data Type Conversion12/1 -> Bus Creator/13  "HealEnable"
  Data Type Conversion13/1 -> Bus Creator/14  "PreestorageFreezeTrigger"
  Data Type Conversion14/1 -> Bus Creator/15  "JumpDownEn"

== system DiagCCaller_TestHarness/DebounceDisabled StartUpComp delay = 1s  ==
  Bus Creator : BusCreator  Inputs=15
  Data Type Conversion{,1..2,9..14} (9 alike) : DataTypeConversion  OutDataTypeStr=boolean
  Data Type Conversion3 : DataTypeConversion  OutDataTypeStr=single
  Data Type Conversion4 : DataTypeConversion  OutDataTypeStr=single
  Data Type Conversion{5..8} (4 alike) : DataTypeConversion  OutDataTypeStr=int16
  Signal Builder : Subsystem  Tag=STV Subsys  LoadFcn=sigbuilder_block('load');  StartFcn=sigbuilder_block('start');  StopFcn=sigbuilder_block('stop');  ClipboardFcn=sigbuilder_block('clipboard');  TreatAsAtomicUnit=on  mask(Sigbuilder block){tuvar=[0:10]}
      mask help: Simulink:masks:SigbuilderBlock_MD
      mask init:
      | if ~strcmp(get_param(bdroot(gcbh),'SimulationStatus'),'stopped') tuvar = sigbuilder_block('maskInit'); end
      settings: CopyFcn=sigbuilder_block('copy');  DeleteFcn=sigbuilder_block('delete');  ModelCloseFcn=sigbuilder_block('modelClose');  PreSaveFcn=sigbuilder_block('preSave');  PauseFcn=sigbuilder_block('pause');  ContinueFcn=sigbuilder_block('continue');  NameChangeFcn=sigbuilder_block('namechange');  OpenFcn=sigbuilder_block('open',[0 30 1152 561.6 ]);  CloseFcn=sigbuilder_block('close');
      mask Display: plot(0, 0, 100, 100,[2, 2, 32, 32, 2], [68, 8, 8, 68, 68],[32, 2], [38, 38], [32, 19, 2],[53, 60, 44], [32, 17, 17, 2],[16, 16, 31, 31]);txt = getActiveGroup(gcbh);text(2, 100, txt,'verticalAlignment', 'top');
  Out1 : Outport
  wires:
  Data Type Conversion14/1 -> Bus Creator/15  "JumpDownEn"
  Data Type Conversion13/1 -> Bus Creator/14  "PreestorageFreezeTrigger"
  Data Type Conversion12/1 -> Bus Creator/13  "HealEnable"
  Data Type Conversion11/1 -> Bus Creator/12  "DiagEnable"
  Data Type Conversion10/1 -> Bus Creator/11  "DiagReset"
  Data Type Conversion9/1 -> Bus Creator/10  "DebounceEn"
  Data Type Conversion8/1 -> Bus Creator/9  "PassCountThd"
  Data Type Conversion7/1 -> Bus Creator/8  "FaultCountThd"
  Data Type Conversion6/1 -> Bus Creator/7  "DownCount"
  Data Type Conversion5/1 -> Bus Creator/6  "UpCount"
  Data Type Conversion3/1 -> Bus Creator/5  "MinValue"
  Data Type Conversion4/1 -> Bus Creator/4  "MaxValue"
  Data Type Conversion2/1 -> Bus Creator/3  "StartupComp"
  Data Type Conversion1/1 -> Bus Creator/2  "DiagInput"
  Data Type Conversion/1 -> Bus Creator/1  "EnableSubsystem"
  Signal Builder/1(EnableSubsystem) -> Data Type Conversion/1
  Signal Builder/15(JumpDownEn) -> Data Type Conversion14/1
  Signal Builder/14(PreestorageFreezeTrigger) -> Data Type Conversion13/1
  Signal Builder/13(HealEnable) -> Data Type Conversion12/1
  Signal Builder/12(DiagEnable) -> Data Type Conversion11/1
  Signal Builder/11(DiagReset) -> Data Type Conversion10/1
  Signal Builder/10(DebounceEn) -> Data Type Conversion9/1
  Signal Builder/9(PassCountThd) -> Data Type Conversion8/1
  Signal Builder/8(FaultCountThd) -> Data Type Conversion7/1
  Signal Builder/7(DownCount) -> Data Type Conversion6/1
  Signal Builder/6(UpCount) -> Data Type Conversion5/1
  Signal Builder/5(MinValue) -> Data Type Conversion3/1
  Signal Builder/4(MaxValue) -> Data Type Conversion4/1
  Signal Builder/3(StartupComp) -> Data Type Conversion2/1
  Signal Builder/2(DiagInput) -> Data Type Conversion1/1
  Bus Creator/1 -> Out1/1
